simulink model "Comparison_SmithPredictor_MIAC_V4"  (R2018b)
settings: Solver=FixedStepDiscrete  StartTime=0.0  StopTime=15  FixedStep=1  RelTol=1e-3
libraries: simulink x2, slident x2
settings Model: Creator=Trips  LastModifiedBy=Trips
settings ConfigComp: PLC_OutputDir=Generated_V4  PLC_TargetIDE=step7  PLC_GenerateReport=off  PLC_LaunchReport=off

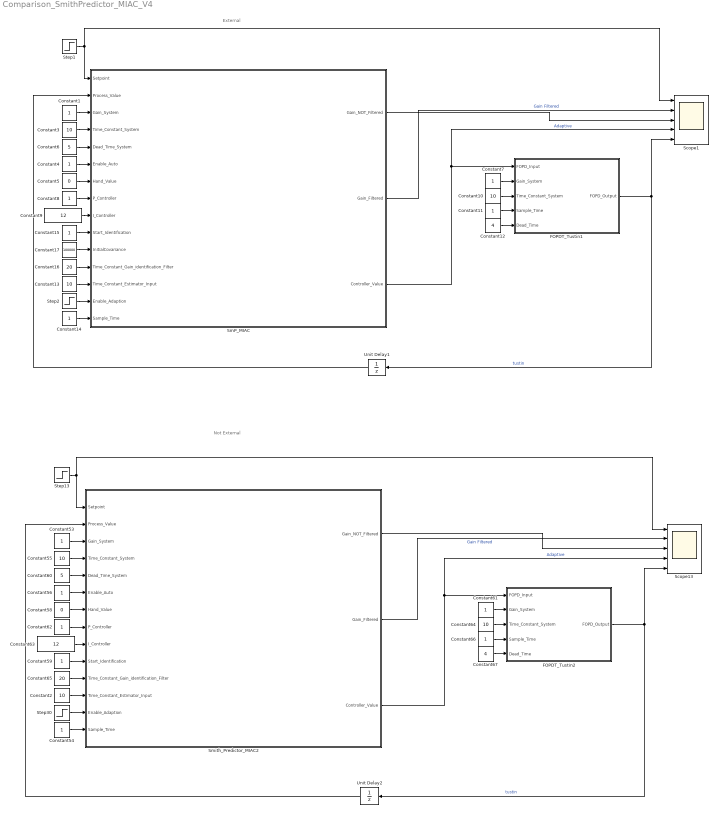
== system Comparison_SmithPredictor_MIAC_V4 ==
  note: External
  note: Not External
  Constant{1,4,7..8,11,14..15,53..54,56,59,61..62,66} (14 alike) : Constant
  Constant{2..3,10,13,55,64} (6 alike) : Constant  Value=10
  Constant12 : Constant  Value=4
  Constant16 : Constant  Value=20
  Constant17 : Constant  Value=100000
  Constant5 : Constant  Value=0
  Constant58 : Constant  Value=0
  Constant6 : Constant  Value=5
  Constant60 : Constant  Value=5
  Constant63 : Constant  Value=12
  Constant65 : Constant  Value=20
  Constant67 : Constant  Value=4
  Constant9 : Constant  Value=12
  FOPDT_Tustin1 : Subsystem  TreatAsAtomicUnit=on  SystemSampleTime=1
  FOPDT_Tustin2 : Subsystem  TreatAsAtomicUnit=on  SystemSampleTime=1
  Scope1 : Scope  NumInputPorts=5
  Scope13 : Scope  NumInputPorts=5
  SmP_MIAC : Subsystem  TreatAsAtomicUnit=on  SystemSampleTime=1
  Smith_Predictor_MIAC2 : Subsystem  TreatAsAtomicUnit=on  SystemSampleTime=1
  Step1 : Step  After=3  SampleTime=0
  Step13 : Step  After=3  SampleTime=0
  Step2 : Step  Time=500  After=0  SampleTime=0
  Step30 : Step  Time=500  After=0  SampleTime=0
  Unit Delay1 : UnitDelay  SampleTime=-1
  Unit Delay2 : UnitDelay  SampleTime=-1
  wires:
  Smith_Predictor_MIAC2/3(Controller_Value) -> Scope13/4, FOPDT_Tustin2/1(FOPD_Input)  "Adaptive"
  Constant56/1 -> Smith_Predictor_MIAC2/6(" Enable_Auto")
  Constant60/1 -> Smith_Predictor_MIAC2/5(Dead_Time_System)
  Constant62/1 -> Smith_Predictor_MIAC2/8(P_Controller)
  Constant55/1 -> Smith_Predictor_MIAC2/4(Time_Constant_System)
  Unit Delay2/1 -> Smith_Predictor_MIAC2/2(Process_Value)
  Constant58/1 -> Smith_Predictor_MIAC2/7(Hand_Value)
  Constant2/1 -> Smith_Predictor_MIAC2/12(Time_Constant_Estimator_Input)
  Constant63/1 -> Smith_Predictor_MIAC2/9(I_Controller)
  Constant65/1 -> Smith_Predictor_MIAC2/11(Time_Constant_Gain_identification_Filter)
  Constant66/1 -> FOPDT_Tustin2/4(Sample_Time)
  Constant61/1 -> FOPDT_Tustin2/2(Gain_System)
  Constant67/1 -> FOPDT_Tustin2/5(" Dead_Time")
  Constant64/1 -> FOPDT_Tustin2/3(Time_Constant_System)
  Step13/1 -> Smith_Predictor_MIAC2/1(Setpoint), Scope13/1
  FOPDT_Tustin2/1(FOPD_Output) -> Scope13/5, Unit Delay2/1  "tustin"
  Smith_Predictor_MIAC2/2(Gain_Filtered) -> Scope13/2  "Gain Filtered"
  Constant54/1 -> Smith_Predictor_MIAC2/14(Sample_Time)
  Constant53/1 -> Smith_Predictor_MIAC2/3(Gain_System)
  Smith_Predictor_MIAC2/1(Gain_NOT_Filtered) -> Scope13/3
  Step30/1 -> Smith_Predictor_MIAC2/13(Enable_Adaption)
  Constant59/1 -> Smith_Predictor_MIAC2/10(Start_Identification)
  SmP_MIAC/1(Gain_NOT_Filtered) -> Scope1/3
  Constant1/1 -> SmP_MIAC/3(Gain_System)
  SmP_MIAC/2(Gain_Filtered) -> Scope1/2  "Gain Filtered"
  Step1/1 -> SmP_MIAC/1(Setpoint), Scope1/1
  Constant10/1 -> FOPDT_Tustin1/3(Time_Constant_System)
  Constant12/1 -> FOPDT_Tustin1/5(" Dead_Time")
  Constant7/1 -> FOPDT_Tustin1/2(Gain_System)
  Constant11/1 -> FOPDT_Tustin1/4(Sample_Time)
  Constant3/1 -> SmP_MIAC/4(Time_Constant_System)
  Constant5/1 -> SmP_MIAC/7(Hand_Value)
  Constant8/1 -> SmP_MIAC/8(P_Controller)
  Unit Delay1/1 -> SmP_MIAC/2(Process_Value)
  Constant6/1 -> SmP_MIAC/5(Dead_Time_System)
  Constant4/1 -> SmP_MIAC/6(" Enable_Auto")
  FOPDT_Tustin1/1(FOPD_Output) -> Scope1/5, Unit Delay1/1  "tustin"
  SmP_MIAC/3(Controller_Value) -> Scope1/4, FOPDT_Tustin1/1(FOPD_Input)  "Adaptive"
  Constant9/1 -> SmP_MIAC/9(I_Controller)
  Step2/1 -> SmP_MIAC/14(Enable_Adaption)
  Constant14/1 -> SmP_MIAC/15(Sample_Time)
  Constant16/1 -> SmP_MIAC/12(Time_Constant_Gain_identification_Filter)
  Constant15/1 -> SmP_MIAC/10(Start_Identification)
  Constant13/1 -> SmP_MIAC/13(Time_Constant_Estimator_Input)
  Constant17/1 -> SmP_MIAC/11(InitialCovariance)

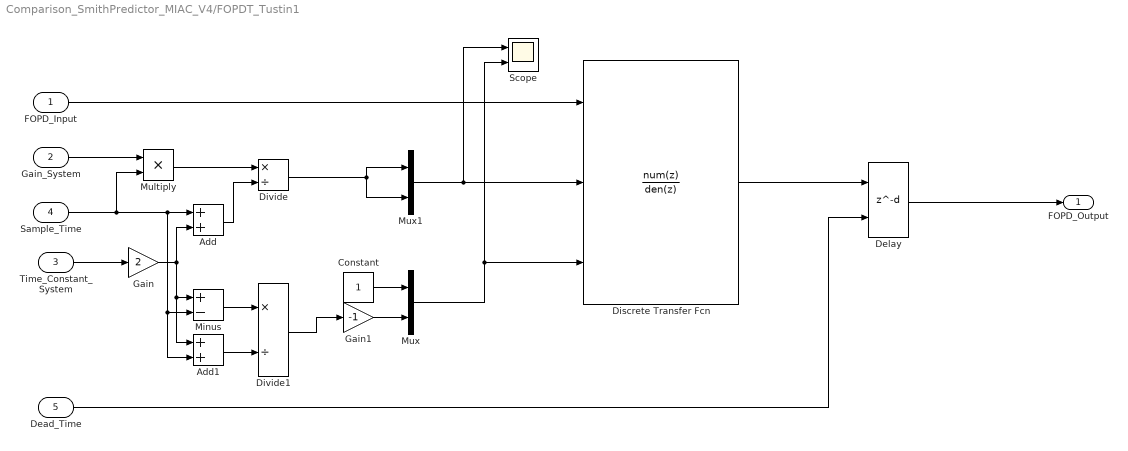
== system Comparison_SmithPredictor_MIAC_V4/FOPDT_Tustin1 ==
  FOPD_Input : Inport
  Gain_System : Inport  Port=2
  Time_Constant_System : Inport  Port=3
  Sample_Time : Inport  Port=4
  " Dead_Time" : Inport  Port=5
  Add : Sum
  Add1 : Sum
  Constant : Constant
  Delay : Delay  DelayLengthSource=Input port  DelayLength=600  DelayLengthUpperLimit=800
      settings: InputPortMap=u0,p1
  Discrete Transfer Fcn : DiscreteTransferFcn  NumeratorSource=Input port  DenominatorSource=Input port  SampleTime=1  a0EqualsOne=on
      settings: InputPortMap=u0,p1,p3
  Divide : Product  Inputs=*/
  Divide1 : Product  Inputs=*/
  Gain : Gain  Gain=2
  Gain1 : Gain  Gain=-1
  Minus : Sum  Inputs=+-
  Multiply : Product
  Mux : Mux  Inputs=2
  Mux1 : Mux  Inputs=2
  Scope : Scope  NumInputPorts=2
  FOPD_Output : Outport
  wires:
  FOPD_Input/1 -> Discrete Transfer Fcn/1
  Discrete Transfer Fcn/1 -> Delay/1
  Mux/1 -> Scope/2, Discrete Transfer Fcn/3
  " Dead_Time"/1 -> Delay/2
  Sample_Time/1 -> Add1/2, Minus/2, Add/1, Multiply/2
  Mux1/1 -> Scope/1, Discrete Transfer Fcn/2
  Time_Constant_System/1 -> Gain/1
  Delay/1 -> FOPD_Output/1
  Gain_System/1 -> Multiply/1
  Multiply/1 -> Divide/1
  Gain/1 -> Add1/1, Minus/1, Add/2
  Add/1 -> Divide/2
  Divide/1 -> Mux1/2, Mux1/1
  Constant/1 -> Mux/1
  Minus/1 -> Divide1/1
  Add1/1 -> Divide1/2
  Divide1/1 -> Gain1/1
  Gain1/1 -> Mux/2

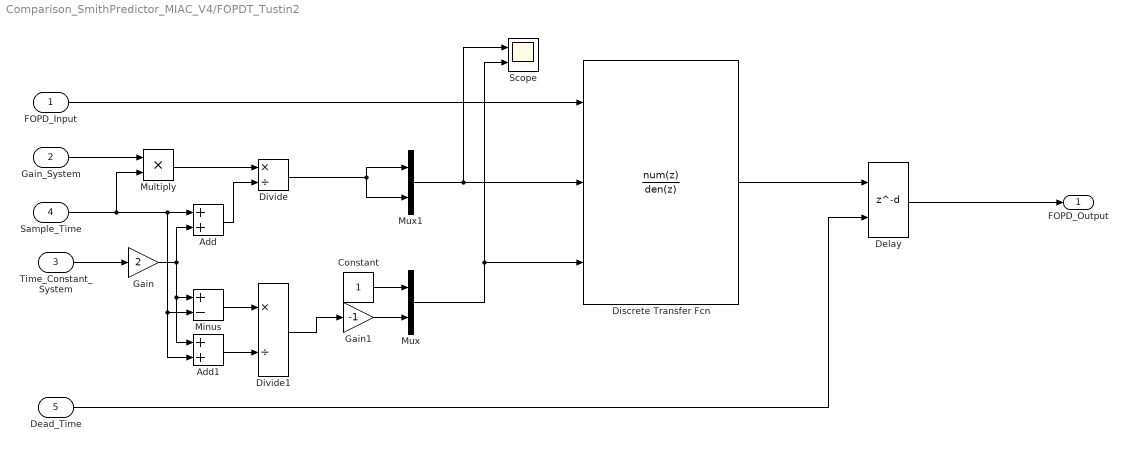
== system Comparison_SmithPredictor_MIAC_V4/FOPDT_Tustin2 ==
  FOPD_Input : Inport
  Gain_System : Inport  Port=2
  Time_Constant_System : Inport  Port=3
  Sample_Time : Inport  Port=4
  " Dead_Time" : Inport  Port=5
  Add : Sum
  Add1 : Sum
  Constant : Constant
  Delay : Delay  DelayLengthSource=Input port  DelayLength=600  DelayLengthUpperLimit=800
      settings: InputPortMap=u0,p1
  Discrete Transfer Fcn : DiscreteTransferFcn  NumeratorSource=Input port  DenominatorSource=Input port  SampleTime=1  a0EqualsOne=on
      settings: InputPortMap=u0,p1,p3
  Divide : Product  Inputs=*/
  Divide1 : Product  Inputs=*/
  Gain : Gain  Gain=2
  Gain1 : Gain  Gain=-1
  Minus : Sum  Inputs=+-
  Multiply : Product
  Mux : Mux  Inputs=2
  Mux1 : Mux  Inputs=2
  Scope : Scope  NumInputPorts=2
  FOPD_Output : Outport
  wires:
  FOPD_Input/1 -> Discrete Transfer Fcn/1
  Discrete Transfer Fcn/1 -> Delay/1
  Mux/1 -> Scope/2, Discrete Transfer Fcn/3
  " Dead_Time"/1 -> Delay/2
  Sample_Time/1 -> Add1/2, Minus/2, Add/1, Multiply/2
  Mux1/1 -> Scope/1, Discrete Transfer Fcn/2
  Time_Constant_System/1 -> Gain/1
  Delay/1 -> FOPD_Output/1
  Gain_System/1 -> Multiply/1
  Multiply/1 -> Divide/1
  Gain/1 -> Add1/1, Minus/1, Add/2
  Add/1 -> Divide/2
  Divide/1 -> Mux1/2, Mux1/1
  Constant/1 -> Mux/1
  Minus/1 -> Divide1/1
  Add1/1 -> Divide1/2
  Divide1/1 -> Gain1/1
  Gain1/1 -> Mux/2

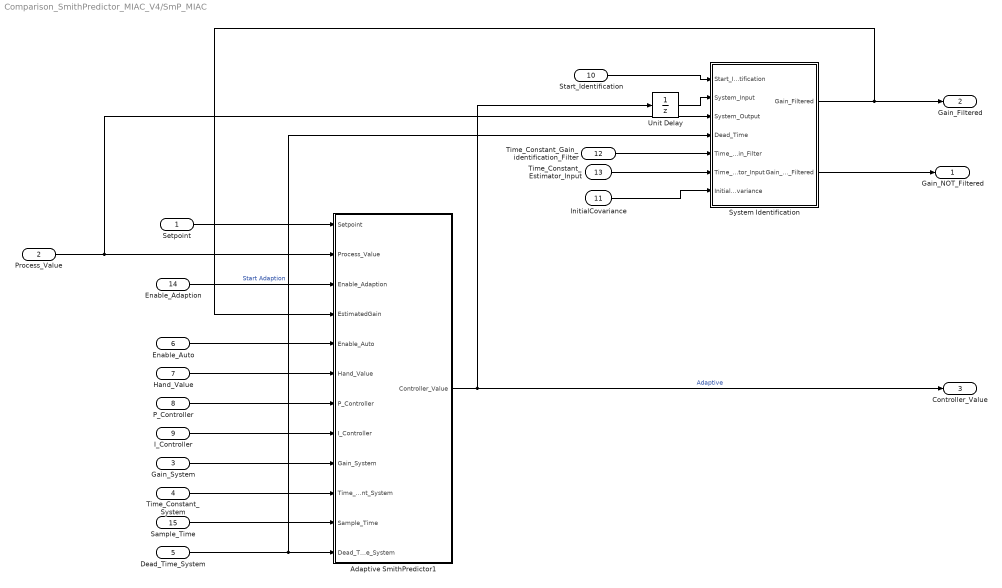
== system Comparison_SmithPredictor_MIAC_V4/SmP_MIAC ==
  Setpoint : Inport
  Process_Value : Inport  Port=2
  Gain_System : Inport  Port=3
  Time_Constant_System : Inport  Port=4
  Dead_Time_System : Inport  Port=5
  " Enable_Auto" : Inport  Port=6
  Hand_Value : Inport  Port=7
  P_Controller : Inport  Port=8
  I_Controller : Inport  Port=9
  Start_Identification : Inport  Port=10  PortDimensions=1  SampleTime=1
  InitialCovariance : Inport  Port=11
  Time_Constant_Gain_identification_Filter : Inport  Port=12
  Time_Constant_Estimator_Input : Inport  Port=13
  Enable_Adaption : Inport  Port=14
  Sample_Time : Inport  Port=15
  Adaptive SmithPredictor1 : Subsystem  TreatAsAtomicUnit=on  SystemSampleTime=1
  System Identification : Subsystem  TreatAsAtomicUnit=on  SystemSampleTime=1
  Unit Delay : UnitDelay
  Gain_NOT_Filtered : Outport
  Gain_Filtered : Outport  Port=2
  Controller_Value : Outport  Port=3
  wires:
  Gain_System/1 -> Adaptive SmithPredictor1/9(Gain_System)
  Dead_Time_System/1 -> Adaptive SmithPredictor1/12(" Dead_Time_System"), System Identification/4(Dead_Time)
  Adaptive SmithPredictor1/1(Controller_Value) -> Unit Delay/1, Controller_Value/1  "Adaptive"
  Time_Constant_System/1 -> Adaptive SmithPredictor1/10(Time_Constant_System)
  P_Controller/1 -> Adaptive SmithPredictor1/7(P_Controller)
  Sample_Time/1 -> Adaptive SmithPredictor1/11(Sample_Time)
  I_Controller/1 -> Adaptive SmithPredictor1/8(I_Controller)
  Enable_Adaption/1 -> Adaptive SmithPredictor1/3(Enable_Adaption)  "Start Adaption"
  System Identification/2(Gain_Not_Filtered) -> Gain_NOT_Filtered/1
  Setpoint/1 -> Adaptive SmithPredictor1/1(Setpoint)
  Start_Identification/1 -> System Identification/1(Start_Identification)
  System Identification/1(Gain_Filtered) -> Gain_Filtered/1, Adaptive SmithPredictor1/4(EstimatedGain)
  " Enable_Auto"/1 -> Adaptive SmithPredictor1/5(Enable_Auto)
  Hand_Value/1 -> Adaptive SmithPredictor1/6(Hand_Value)
  Process_Value/1 -> System Identification/3(System_Output), Adaptive SmithPredictor1/2(Process_Value)
  Unit Delay/1 -> System Identification/2(System_Input)
  Time_Constant_Gain_identification_Filter/1 -> System Identification/5(Time_Constant_Gain_Filter)
  Time_Constant_Estimator_Input/1 -> System Identification/6(Time_Constant_Estimator_Input)
  InitialCovariance/1 -> System Identification/7(InitialCovariance)

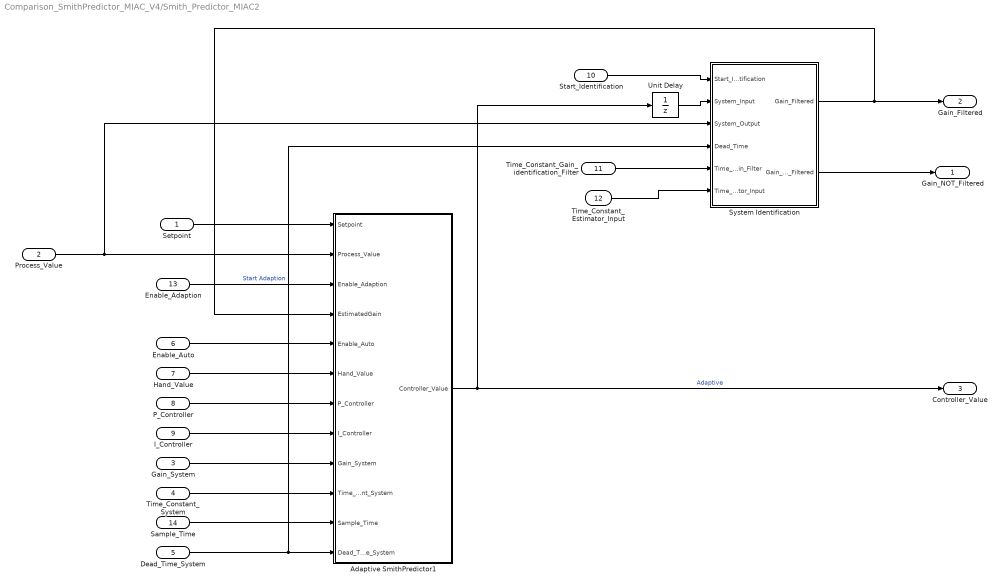
== system Comparison_SmithPredictor_MIAC_V4/Smith_Predictor_MIAC2 ==
  Setpoint : Inport
  Process_Value : Inport  Port=2
  Gain_System : Inport  Port=3
  Time_Constant_System : Inport  Port=4
  Dead_Time_System : Inport  Port=5
  " Enable_Auto" : Inport  Port=6
  Hand_Value : Inport  Port=7
  P_Controller : Inport  Port=8
  I_Controller : Inport  Port=9
  Start_Identification : Inport  Port=10  PortDimensions=1  SampleTime=1
  Time_Constant_Gain_identification_Filter : Inport  Port=11
  Time_Constant_Estimator_Input : Inport  Port=12
  Enable_Adaption : Inport  Port=13
  Sample_Time : Inport  Port=14
  Adaptive SmithPredictor1 : Subsystem  TreatAsAtomicUnit=on  SystemSampleTime=1
  System Identification : Subsystem  TreatAsAtomicUnit=on  SystemSampleTime=1
  Unit Delay : UnitDelay
  Gain_NOT_Filtered : Outport
  Gain_Filtered : Outport  Port=2
  Controller_Value : Outport  Port=3
  wires:
  Gain_System/1 -> Adaptive SmithPredictor1/9(Gain_System)
  Dead_Time_System/1 -> Adaptive SmithPredictor1/12(" Dead_Time_System"), System Identification/4(Dead_Time)
  Adaptive SmithPredictor1/1(Controller_Value) -> Unit Delay/1, Controller_Value/1  "Adaptive"
  Time_Constant_System/1 -> Adaptive SmithPredictor1/10(Time_Constant_System)
  P_Controller/1 -> Adaptive SmithPredictor1/7(P_Controller)
  Sample_Time/1 -> Adaptive SmithPredictor1/11(Sample_Time)
  I_Controller/1 -> Adaptive SmithPredictor1/8(I_Controller)
  Enable_Adaption/1 -> Adaptive SmithPredictor1/3(Enable_Adaption)  "Start Adaption"
  System Identification/2(Gain_Not_Filtered) -> Gain_NOT_Filtered/1
  Setpoint/1 -> Adaptive SmithPredictor1/1(Setpoint)
  Start_Identification/1 -> System Identification/1(Start_Identification)
  System Identification/1(Gain_Filtered) -> Gain_Filtered/1, Adaptive SmithPredictor1/4(EstimatedGain)
  " Enable_Auto"/1 -> Adaptive SmithPredictor1/5(Enable_Auto)
  Hand_Value/1 -> Adaptive SmithPredictor1/6(Hand_Value)
  Process_Value/1 -> System Identification/3(System_Output), Adaptive SmithPredictor1/2(Process_Value)
  Unit Delay/1 -> System Identification/2(System_Input)
  Time_Constant_Gain_identification_Filter/1 -> System Identification/5(Time_Constant_Gain_Filter)
  Time_Constant_Estimator_Input/1 -> System Identification/6(Time_Constant_Estimator_Input)

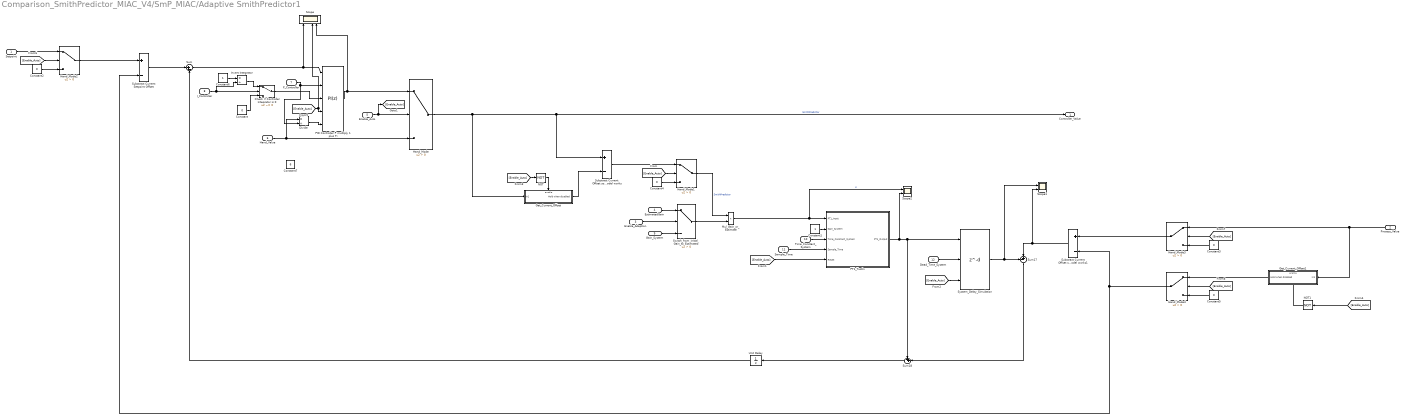
== system Comparison_SmithPredictor_MIAC_V4/SmP_MIAC/Adaptive SmithPredictor1 ==
  Setpoint : Inport
  Process_Value : Inport  Port=2
  Enable_Adaption : Inport  Port=3
  EstimatedGain : Inport  Port=4
  Enable_Auto : Inport  Port=5
  Hand_Value : Inport  Port=6
  P_Controller : Inport  Port=7
  I_Controller : Inport  Port=8
  Gain_System : Inport  Port=9
  Time_Constant_System : Inport  Port=10
  Sample_Time : Inport  Port=11
  " Dead_Time_System" : Inport  Port=12
  Check if Controller Integrator is 0 : Switch  Criteria=u2 ~= 0
  Constant{,2..5} (5 alike) : Constant  Value=0
  Constant1 : Constant
  Constant6 : Constant
  Constant7 : Constant  Value=6
  Divide : Product  Inputs=*/
  Get_Current_Offset : Subsystem
  Get_Current_Offset1 : Subsystem
  Hand_Mode{,1..4} (5 alike) : Switch  Criteria=u2 > Threshold
  Invert Integrator : Product  Inputs=*/
  Mul_Gain_or_Estimate : Product
  NOT : Logic  Operator=NOT  IconShape=distinctive  AllPortsSameDT=off  OutDataTypeStr=boolean
  NOT1 : Logic  Operator=NOT  IconShape=distinctive  AllPortsSameDT=off  OutDataTypeStr=boolean
  "PID Controller P multiply 1 plus Ti " : simulink/Continuous/PID Controller  Controller=PI  Form=Ideal  TimeDomain=Discrete-time  SampleTime=1  IntegratorMethod=Forward Euler  FilterMethod=Forward Euler  ControllerParametersSource=external  P=3.04732259067536  I=0.00445689106465138  D=118.272348286844  UseFilter=on  N=0.00420306193364532  TunerSelectOption=Transfer Function Based (PID Tuner App)  InitialConditionSource=external  InitialConditionForIntegrator=0  InitialConditionForFilter=0  DifferentiatorICPrevScaledInput=0  ExternalReset=rising  TrackingMode=off  Kt=1  LimitOutput=on  UpperSaturationLimit=100  LowerSaturationLimit=0  LinearizeAsGain=on  AntiWindupMode=none  Kb=1  POutMin=[]  POutMax=[]  IOutMin=[]  IOutMax=[]  DOutMin=[]  DOutMax=[]  NOutMin=[]  NOutMax=[]  SumOutMin=[]  SumOutMax=[]  SaturationOutMin=[]  SaturationOutMax=[]  PParamMin=[]  PParamMax=[]  IParamMin=[]  IParamMax=[]  DParamMin=[]  DParamMax=[]  NParamMin=[]  NParamMax=[]  KbParamMin=[]  KbParamMax=[]  KtParamMin=[]  KtParamMax=[]  KbOutMin=[]  KbOutMax=[]  KtOutMin=[]  KtOutMax=[]  IntegratorOutMin=[]  IntegratorOutMax=[]  FilterOutMin=[]  FilterOutMax=[]  SumI1OutMin=[]  SumI1OutMax=[]  SumI2OutMin=[]  SumI2OutMax=[]  SumI3OutMin=[]  SumI3OutMax=[]  SumI4OutMin=[]  SumI4OutMax=[]  SumDOutMin=[]  SumDOutMax=[]  DifferentiatorOutMin=[]  DifferentiatorOutMax=[]  FilterDiffOutCoefMin=[]  FilterDiffOutCoefMax=[]  ReciprocalOutMin=[]  ReciprocalOutMax=[]  SumDenOutMin=[]  SumDenOutMax=[]  SumNumOutMin=[]  SumNumOutMax=[]  DivideOutMin=[]  DivideOutMax=[]  IntegratorContinuousStateAttributes=''  IntegratorStateMustResolveToSignalObject=off  IntegratorRTWStateStorageClass=Auto  FilterContinuousStateAttributes=''  FilterStateMustResolveToSignalObject=off  FilterRTWStateStorageClass=Auto  ParallelPVariant=Passthrough  IdealPVariant=ExternalParameters  IVariant=ExternalParameters  DVariant=Disabled  IntegratorVariant=Discrete  SatVariant=Enabled  AWVariant=Passthrough  PCopyVariant=Disabled  TRVariant=Disabled  FdbkBlocksVariant=Forward  IdealPFdbkVariant=Disabled  SatFdbkVariant=Disabled  DerivativeFilterVariant=Disabled  NVariant=Disabled  NCopyVariant=Disabled_SignalSpec  FilterICVariant=Disabled  IntegratorICVariant=ExternalICs  ExternalResetVariant=ExternalReset  TRSumVariant=Passthrough  SumFdbkVariant=Disabled  SumVariant=Sum_PI
  PT1_Tustin : Subsystem  TreatAsAtomicUnit=on  SystemSampleTime=1
  Scope : Scope  NumInputPorts=4
  Scope1 : Scope  NumInputPorts=2
  Scope2 : Scope  NumInputPorts=2
  Substract Current Offset so that the linearised model works : Sum  Inputs=+-
  Substract Current Offset so that the linearised model works1 : Sum  Inputs=+-
  Substract Current Setpoint Offset : Sum  Inputs=+-
  Sum : Sum  Inputs=|+-
  Sum17 : Sum  Inputs=-+|
  Sum18 : Sum  Inputs=++|
  Switch_from_initial_Gain_to_Estimated : Switch  Criteria=u2 > Threshold
  System_Delay_Simulation : Delay  DelayLengthSource=Input port  DelayLength=600  DelayLengthUpperLimit=900  ExternalReset=Rising  SampleTime=1
      settings: InputPortMap=u0,p1,r5
  Unit Delay : UnitDelay
  Controller_Value : Outport
  wires:
  Substract Current Setpoint Offset/1 -> Sum/1
  Sum/1 -> "PID Controller P multiply 1 plus Ti "/1, Scope/1
  Hand_Mode/1 -> Get_Current_Offset/1(In1), Controller_Value/1, Substract Current Offset so that the linearised model works/1  "SmithPredictor"
  Substract Current Offset so that the linearised model works1/1 -> Scope1/2, Sum17/2
  PT1_Tustin/1(PT1_Output) -> Scope2/2, Sum18/1, System_Delay_Simulation/1
  System_Delay_Simulation/1 -> Scope1/1, Sum17/1
  Sum17/1 -> Sum18/2
  Mul_Gain_or_Estimate/1 -> Scope2/1, PT1_Tustin/1(PT1_Input)  "U"
  Switch_from_initial_Gain_to_Estimated/1 -> Mul_Gain_or_Estimate/2
  "PID Controller P multiply 1 plus Ti "/1 -> Hand_Mode/1, Scope/4
  Hand_Value/1 -> Divide/1, Hand_Mode/3
  Enable_Auto/1 -> [Enable_Auto], Hand_Mode/2
  P_Controller/1 -> "PID Controller P multiply 1 plus Ti "/2, Divide/2
  Check if Controller Integrator is 0/1 -> "PID Controller P multiply 1 plus Ti "/3
  " Dead_Time_System"/1 -> System_Delay_Simulation/2
  Gain_System/1 -> Switch_from_initial_Gain_to_Estimated/3
  Enable_Adaption/1 -> Switch_from_initial_Gain_to_Estimated/2
  EstimatedGain/1 -> Switch_from_initial_Gain_to_Estimated/1
  [Enable_Auto] -> Hand_Mode1/2
  Hand_Mode1/1 -> Mul_Gain_or_Estimate/1  "SmithPredictor"
  Constant4/1 -> Hand_Mode1/3
  [Enable_Auto] -> PT1_Tustin/5(Reset)
  [Enable_Auto] -> System_Delay_Simulation/3
  Substract Current Offset so that the linearised model works/1 -> Hand_Mode1/1
  Get_Current_Offset/1(Hold when disabled) -> Substract Current Offset so that the linearised model works/2
  [Enable_Auto] -> NOT/1
  NOT/1 -> Get_Current_Offset/Enable
  Sum18/1 -> Unit Delay/1
  Hand_Mode2/1 -> Substract Current Setpoint Offset/1
  NOT1/1 -> Get_Current_Offset1/Enable
  [Enable_Auto] -> NOT1/1
  Hand_Mode4/1 -> Substract Current Setpoint Offset/2, Substract Current Offset so that the linearised model works1/2
  Setpoint/1 -> Hand_Mode2/1
  [Enable_Auto] -> Hand_Mode2/2
  Constant2/1 -> Hand_Mode2/3
  Process_Value/1 -> Get_Current_Offset1/1(In1), Hand_Mode3/1
  [Enable_Auto] -> Hand_Mode3/2
  Constant3/1 -> Hand_Mode3/3
  Hand_Mode3/1 -> Substract Current Offset so that the linearised model works1/1
  Constant5/1 -> Hand_Mode4/3
  [Enable_Auto] -> Hand_Mode4/2
  Get_Current_Offset1/1(Hold when disabled) -> Hand_Mode4/1
  Time_Constant_System/1 -> PT1_Tustin/3(Time_Constant_System)
  Constant1/1 -> PT1_Tustin/2(Gain_System)
  Sample_Time/1 -> PT1_Tustin/4(Sample_Time)
  I_Controller/1 -> Check if Controller Integrator is 0/2, Invert Integrator/2
  Constant/1 -> Check if Controller Integrator is 0/3
  Invert Integrator/1 -> Check if Controller Integrator is 0/1
  Constant6/1 -> Invert Integrator/1
  Unit Delay/1 -> Sum/2
  [Enable_Auto] -> Scope/3, "PID Controller P multiply 1 plus Ti "/4
  Divide/1 -> "PID Controller P multiply 1 plus Ti "/5

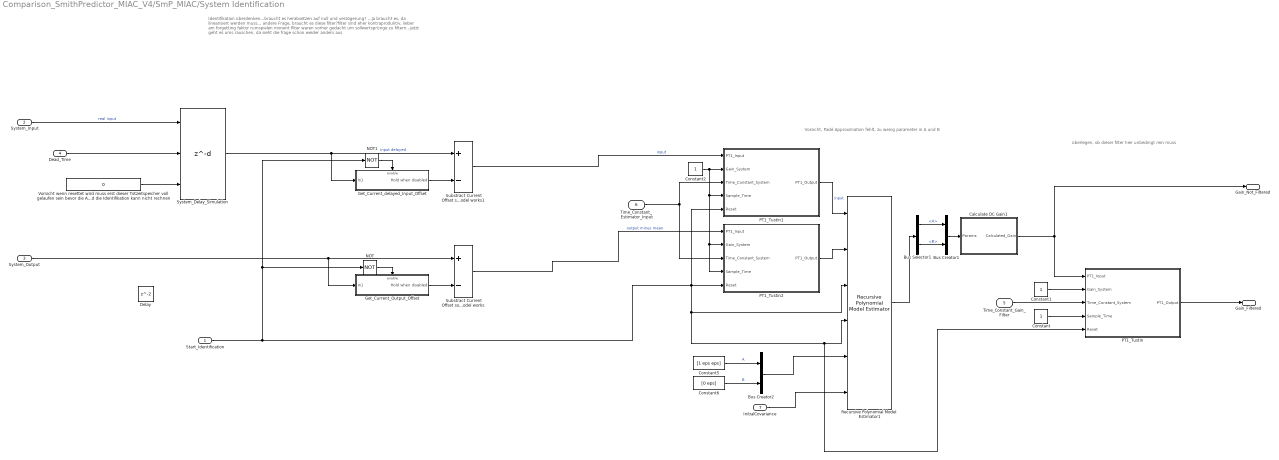
== system Comparison_SmithPredictor_MIAC_V4/SmP_MIAC/System Identification ==
  note: Vorsicht, Padé Approximation fehlt, zu wenig parameter in A und B
  note: überlegen, ob dieser filter hier unbedingt rein muss
  note: Identifikation überdenken...braucht es herabsetzen auf null und verzögerung?
      | ...ja braucht es, da linearisiert werden muss...
      |
      | andere Frage, braucht es diese filter?filter sind eher kontraproduktiv, lieber am forgetting faktor rumspielen
      | monent fliter waren vorher gedacht um sollwertsprünge zu filtern...jetzt geht es ums rauschen, da sieht die frage schon weider anders aus
  Start_Identification : Inport  SampleTime=1
  System_Input : Inport  Port=2
  System_Output : Inport  Port=3  SampleTime=1
  Dead_Time : Inport  Port=4
  Time_Constant_Gain_Filter : Inport  Port=5
  Time_Constant_Estimator_Input : Inport  Port=6
  InitialCovariance : Inport  Port=7  SampleTime=1
  Bus Creator1 : BusCreator  Inputs=2
  Bus Creator2 : BusCreator  Inputs=2
  Bus Selector1 : BusSelector  OutputSignals=A,B
  Calculate DC Gain1 : Subsystem  TreatAsAtomicUnit=on  SystemSampleTime=1
  Constant : Constant
  Constant1 : Constant
  Constant2 : Constant
  Constant5 : Constant  Value=[1 eps eps]  VectorParams1D=off
  Constant6 : Constant  Value=[0 eps]  VectorParams1D=off
  Delay : Delay
  Get_Current_Output_Offset : Subsystem
  Get_Current_delayed_Input_Offset : Subsystem
  NOT : Logic  Operator=NOT  IconShape=distinctive  AllPortsSameDT=off  OutDataTypeStr=boolean
  NOT1 : Logic  Operator=NOT  IconShape=distinctive  AllPortsSameDT=off  OutDataTypeStr=boolean
  PT1_Tustin : Subsystem  TreatAsAtomicUnit=on  SystemSampleTime=1
  PT1_Tustin1 : Subsystem  TreatAsAtomicUnit=on  SystemSampleTime=1
  PT1_Tustin2 : Subsystem  TreatAsAtomicUnit=on  SystemSampleTime=1
  Recursive Polynomial Model Estimator1 : slident/Estimators/Recursive Polynomial Model Estimator  ModelStructure=ARX  InitialEstimateSource=External  A0=2  B0=1  C0=1  D0=1  F0=1  nk=1  P0=10  InitialInputs=0  InitialOutputs=0  History=Infinite  WindowLength=2000  EstimationMethod=Forgetting Factor  AdaptationParameter=1  HasTimeVaryingAdaptationParameter=off  NormalizationBias=eps  OutputError=off  OutputP=off  AddEnablePort=on  ExternalReset=Rising  InputProcessing=Sample-based  Ts=1
      settings: SourceProductName=System Identification Toolbox  SourceProductBaseCode=ID
  Substract Current Offset so that the linearised model works : Sum  Inputs=+-
  Substract Current Offset so that the linearised model works1 : Sum  Inputs=+-
  System_Delay_Simulation : Delay  DelayLengthSource=Input port  DelayLength=600  DelayLengthUpperLimit=900  ExternalReset=Rising  SampleTime=1
      settings: InputPortMap=u0,p1,r5
  Vorsicht wenn resettet wird muss erst dieser Totzeitspeicher voll gelaufen sein bevor die Adaption starten darf Sonst kommt heir immer 0 raus und die Identifikation kann nicht rechnen : Constant  Value=0
  Gain_Filtered : Outport
  Gain_Not_Filtered : Outport  Port=2
  wires:
  Recursive Polynomial Model Estimator1/1 -> Bus Selector1/1
  Substract Current Offset so that the linearised model works1/1 -> PT1_Tustin1/1(PT1_Input)  "input"
  Bus Creator1/1 -> Calculate DC Gain1/1(Params)
  Bus Selector1/1 -> Bus Creator1/1  "<A>"
  Bus Selector1/2 -> Bus Creator1/2  "<B>"
  Substract Current Offset so that the linearised model works/1 -> PT1_Tustin2/1(PT1_Input)  "output minus mean"
  NOT/1 -> Get_Current_Output_Offset/Enable
  Get_Current_Output_Offset/1(Hold when disabled) -> Substract Current Offset so that the linearised model works/2
  System_Output/1 -> Get_Current_Output_Offset/1(In1), Substract Current Offset so that the linearised model works/1
  Get_Current_delayed_Input_Offset/1(Hold when disabled) -> Substract Current Offset so that the linearised model works1/2
  NOT1/1 -> Get_Current_delayed_Input_Offset/Enable
  PT1_Tustin/1(PT1_Output) -> Gain_Filtered/1
  System_Input/1 -> System_Delay_Simulation/1  "real input"
  Vorsicht wenn resettet wird muss erst dieser Totzeitspeicher voll gelaufen sein bevor die Adaption starten darf Sonst kommt heir immer 0 raus und die Identifikation kann nicht rechnen/1 -> System_Delay_Simulation/3
  Dead_Time/1 -> System_Delay_Simulation/2
  System_Delay_Simulation/1 -> Substract Current Offset so that the linearised model works1/1, Get_Current_delayed_Input_Offset/1(In1)  "input delayed"
  Calculate DC Gain1/1(Calculated_Gain) -> PT1_Tustin/1(PT1_Input), Gain_Not_Filtered/1
  Start_Identification/1 -> NOT/1, NOT1/1, PT1_Tustin2/5(Reset), Recursive Polynomial Model Estimator1/3, PT1_Tustin/5(Reset), Recursive Polynomial Model Estimator1/4, PT1_Tustin1/5(Reset)
  Constant/1 -> PT1_Tustin/4(Sample_Time)
  Constant1/1 -> PT1_Tustin/2(Gain_System)
  Time_Constant_Gain_Filter/1 -> PT1_Tustin/3(Time_Constant_System)
  PT1_Tustin1/1(PT1_Output) -> Recursive Polynomial Model Estimator1/1  "input"
  PT1_Tustin2/1(PT1_Output) -> Recursive Polynomial Model Estimator1/2
  Constant2/1 -> PT1_Tustin1/2(Gain_System), PT1_Tustin2/2(Gain_System), PT1_Tustin2/4(Sample_Time), PT1_Tustin1/4(Sample_Time)
  Time_Constant_Estimator_Input/1 -> PT1_Tustin2/3(Time_Constant_System), PT1_Tustin1/3(Time_Constant_System)
  Constant6/1 -> Bus Creator2/2  "B"
  Constant5/1 -> Bus Creator2/1  "A"
  Bus Creator2/1 -> Recursive Polynomial Model Estimator1/5
  InitialCovariance/1 -> Recursive Polynomial Model Estimator1/6

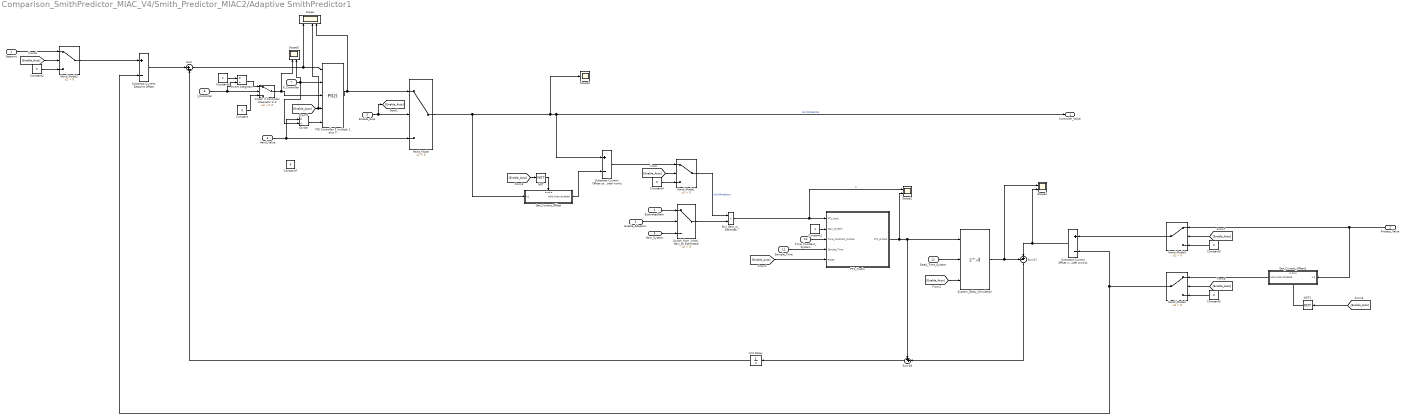
== system Comparison_SmithPredictor_MIAC_V4/Smith_Predictor_MIAC2/Adaptive SmithPredictor1 ==
  Setpoint : Inport
  Process_Value : Inport  Port=2
  Enable_Adaption : Inport  Port=3
  EstimatedGain : Inport  Port=4
  Enable_Auto : Inport  Port=5
  Hand_Value : Inport  Port=6
  P_Controller : Inport  Port=7
  I_Controller : Inport  Port=8
  Gain_System : Inport  Port=9
  Time_Constant_System : Inport  Port=10
  Sample_Time : Inport  Port=11
  " Dead_Time_System" : Inport  Port=12
  Check if Controller Integrator is 0 : Switch  Criteria=u2 ~= 0
  Constant{,2..5} (5 alike) : Constant  Value=0
  Constant1 : Constant
  Constant6 : Constant
  Constant7 : Constant  Value=6
  Divide : Product  Inputs=*/
  Get_Current_Offset : Subsystem
  Get_Current_Offset1 : Subsystem
  Hand_Mode{,1..4} (5 alike) : Switch  Criteria=u2 > Threshold
  Invert Integrator : Product  Inputs=*/
  Mul_Gain_or_Estimate : Product
  NOT : Logic  Operator=NOT  IconShape=distinctive  AllPortsSameDT=off  OutDataTypeStr=boolean
  NOT1 : Logic  Operator=NOT  IconShape=distinctive  AllPortsSameDT=off  OutDataTypeStr=boolean
  "PID Controller P multiply 1 plus Ti " : simulink/Continuous/PID Controller  Controller=PI  Form=Ideal  TimeDomain=Discrete-time  SampleTime=1  IntegratorMethod=Forward Euler  FilterMethod=Forward Euler  ControllerParametersSource=external  P=3.04732259067536  I=0.00445689106465138  D=118.272348286844  UseFilter=on  N=0.00420306193364532  TunerSelectOption=Transfer Function Based (PID Tuner App)  InitialConditionSource=external  InitialConditionForIntegrator=0  InitialConditionForFilter=0  DifferentiatorICPrevScaledInput=0  ExternalReset=rising  TrackingMode=off  Kt=1  LimitOutput=on  UpperSaturationLimit=100  LowerSaturationLimit=0  LinearizeAsGain=on  AntiWindupMode=none  Kb=1  POutMin=[]  POutMax=[]  IOutMin=[]  IOutMax=[]  DOutMin=[]  DOutMax=[]  NOutMin=[]  NOutMax=[]  SumOutMin=[]  SumOutMax=[]  SaturationOutMin=[]  SaturationOutMax=[]  PParamMin=[]  PParamMax=[]  IParamMin=[]  IParamMax=[]  DParamMin=[]  DParamMax=[]  NParamMin=[]  NParamMax=[]  KbParamMin=[]  KbParamMax=[]  KtParamMin=[]  KtParamMax=[]  KbOutMin=[]  KbOutMax=[]  KtOutMin=[]  KtOutMax=[]  IntegratorOutMin=[]  IntegratorOutMax=[]  FilterOutMin=[]  FilterOutMax=[]  SumI1OutMin=[]  SumI1OutMax=[]  SumI2OutMin=[]  SumI2OutMax=[]  SumI3OutMin=[]  SumI3OutMax=[]  SumI4OutMin=[]  SumI4OutMax=[]  SumDOutMin=[]  SumDOutMax=[]  DifferentiatorOutMin=[]  DifferentiatorOutMax=[]  FilterDiffOutCoefMin=[]  FilterDiffOutCoefMax=[]  ReciprocalOutMin=[]  ReciprocalOutMax=[]  SumDenOutMin=[]  SumDenOutMax=[]  SumNumOutMin=[]  SumNumOutMax=[]  DivideOutMin=[]  DivideOutMax=[]  IntegratorContinuousStateAttributes=''  IntegratorStateMustResolveToSignalObject=off  IntegratorRTWStateStorageClass=Auto  FilterContinuousStateAttributes=''  FilterStateMustResolveToSignalObject=off  FilterRTWStateStorageClass=Auto  ParallelPVariant=Passthrough  IdealPVariant=ExternalParameters  IVariant=ExternalParameters  DVariant=Disabled  IntegratorVariant=Discrete  SatVariant=Enabled  AWVariant=Passthrough  PCopyVariant=Disabled  TRVariant=Disabled  FdbkBlocksVariant=Forward  IdealPFdbkVariant=Disabled  SatFdbkVariant=Disabled  DerivativeFilterVariant=Disabled  NVariant=Disabled  NCopyVariant=Disabled_SignalSpec  FilterICVariant=Disabled  IntegratorICVariant=ExternalICs  ExternalResetVariant=ExternalReset  TRSumVariant=Passthrough  SumFdbkVariant=Disabled  SumVariant=Sum_PI
  PT1_Tustin : Subsystem  TreatAsAtomicUnit=on  SystemSampleTime=1
  Scope : Scope  NumInputPorts=4
  Scope1 : Scope  NumInputPorts=2
  Scope2 : Scope  NumInputPorts=2
  Scope3 : Scope  NumInputPorts=2
  Scope4 : Scope
  Substract Current Offset so that the linearised model works : Sum  Inputs=+-
  Substract Current Offset so that the linearised model works1 : Sum  Inputs=+-
  Substract Current Setpoint Offset : Sum  Inputs=+-
  Sum : Sum  Inputs=|+-
  Sum17 : Sum  Inputs=-+|
  Sum18 : Sum  Inputs=++|
  Switch_from_initial_Gain_to_Estimated : Switch  Criteria=u2 > Threshold
  System_Delay_Simulation : Delay  DelayLengthSource=Input port  DelayLength=600  DelayLengthUpperLimit=800  ExternalReset=Rising  SampleTime=1
      settings: InputPortMap=u0,p1,r5
  Unit Delay : UnitDelay
  Controller_Value : Outport
  wires:
  Substract Current Setpoint Offset/1 -> Sum/1
  Sum/1 -> "PID Controller P multiply 1 plus Ti "/1, Scope/1
  Hand_Mode/1 -> Get_Current_Offset/1(In1), Scope4/1, Controller_Value/1, Substract Current Offset so that the linearised model works/1  "SmithPredictor"
  Substract Current Offset so that the linearised model works1/1 -> Scope1/2, Sum17/2
  PT1_Tustin/1(PT1_Output) -> Scope2/2, Sum18/1, System_Delay_Simulation/1
  System_Delay_Simulation/1 -> Scope1/1, Sum17/1
  Sum17/1 -> Sum18/2
  Mul_Gain_or_Estimate/1 -> Scope2/1, PT1_Tustin/1(PT1_Input)  "U"
  Switch_from_initial_Gain_to_Estimated/1 -> Mul_Gain_or_Estimate/2
  "PID Controller P multiply 1 plus Ti "/1 -> Hand_Mode/1, Scope/4
  Hand_Value/1 -> Divide/1, Hand_Mode/3
  Enable_Auto/1 -> [Enable_Auto], Hand_Mode/2
  P_Controller/1 -> "PID Controller P multiply 1 plus Ti "/2, Scope3/2, Divide/2
  Check if Controller Integrator is 0/1 -> Scope3/1, "PID Controller P multiply 1 plus Ti "/3
  " Dead_Time_System"/1 -> System_Delay_Simulation/2
  Gain_System/1 -> Switch_from_initial_Gain_to_Estimated/3
  Enable_Adaption/1 -> Switch_from_initial_Gain_to_Estimated/2
  EstimatedGain/1 -> Switch_from_initial_Gain_to_Estimated/1
  [Enable_Auto] -> Hand_Mode1/2
  Hand_Mode1/1 -> Mul_Gain_or_Estimate/1  "SmithPredictor"
  Constant4/1 -> Hand_Mode1/3
  [Enable_Auto] -> PT1_Tustin/5(Reset)
  [Enable_Auto] -> System_Delay_Simulation/3
  Substract Current Offset so that the linearised model works/1 -> Hand_Mode1/1
  Get_Current_Offset/1(Hold when disabled) -> Substract Current Offset so that the linearised model works/2
  [Enable_Auto] -> NOT/1
  NOT/1 -> Get_Current_Offset/Enable
  Sum18/1 -> Unit Delay/1
  Hand_Mode2/1 -> Substract Current Setpoint Offset/1
  NOT1/1 -> Get_Current_Offset1/Enable
  [Enable_Auto] -> NOT1/1
  Hand_Mode4/1 -> Substract Current Setpoint Offset/2, Substract Current Offset so that the linearised model works1/2
  Setpoint/1 -> Hand_Mode2/1
  [Enable_Auto] -> Hand_Mode2/2
  Constant2/1 -> Hand_Mode2/3
  Process_Value/1 -> Get_Current_Offset1/1(In1), Hand_Mode3/1
  [Enable_Auto] -> Hand_Mode3/2
  Constant3/1 -> Hand_Mode3/3
  Hand_Mode3/1 -> Substract Current Offset so that the linearised model works1/1
  Constant5/1 -> Hand_Mode4/3
  [Enable_Auto] -> Hand_Mode4/2
  Get_Current_Offset1/1(Hold when disabled) -> Hand_Mode4/1
  Time_Constant_System/1 -> PT1_Tustin/3(Time_Constant_System)
  Constant1/1 -> PT1_Tustin/2(Gain_System)
  Sample_Time/1 -> PT1_Tustin/4(Sample_Time)
  I_Controller/1 -> Check if Controller Integrator is 0/2, Invert Integrator/2
  Constant/1 -> Check if Controller Integrator is 0/3
  Invert Integrator/1 -> Check if Controller Integrator is 0/1
  Constant6/1 -> Invert Integrator/1
  Unit Delay/1 -> Sum/2
  [Enable_Auto] -> Scope/3, "PID Controller P multiply 1 plus Ti "/4
  Divide/1 -> "PID Controller P multiply 1 plus Ti "/5

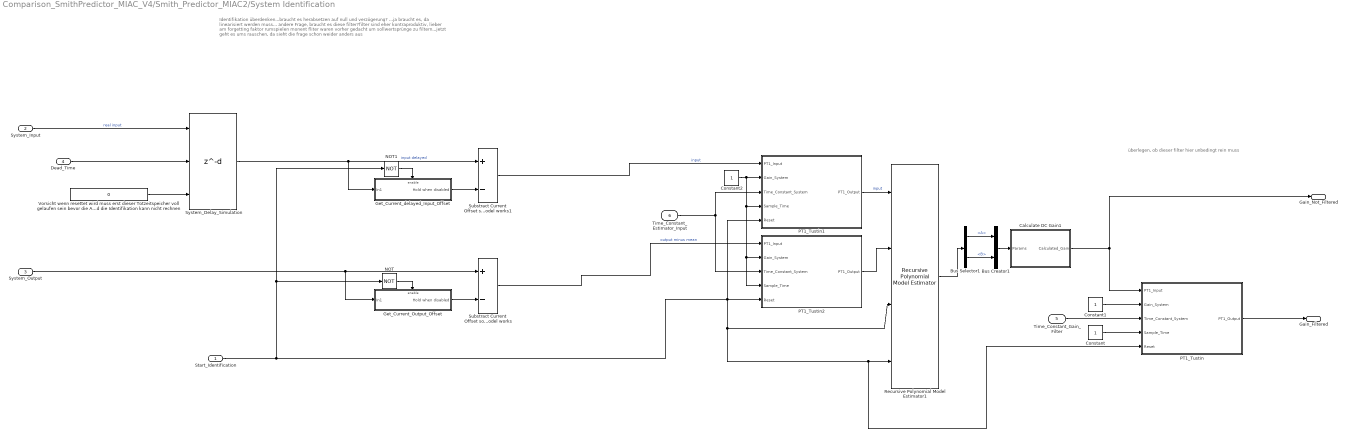
== system Comparison_SmithPredictor_MIAC_V4/Smith_Predictor_MIAC2/System Identification ==
  note: überlegen, ob dieser filter hier unbedingt rein muss
  note: Identifikation überdenken...braucht es herabsetzen auf null und verzögerung?
      | ...ja braucht es, da linearisiert werden muss...
      |
      | andere Frage, braucht es diese filter?filter sind eher kontraproduktiv, lieber am forgetting faktor rumspielen
      | monent fliter waren vorher gedacht um sollwertsprünge zu filtern...jetzt geht es ums rauschen, da sieht die frage schon weider anders aus
  Start_Identification : Inport  SampleTime=1
  System_Input : Inport  Port=2
  System_Output : Inport  Port=3  SampleTime=1
  Dead_Time : Inport  Port=4
  Time_Constant_Gain_Filter : Inport  Port=5
  Time_Constant_Estimator_Input : Inport  Port=6
  Bus Creator1 : BusCreator  Inputs=2
  Bus Selector1 : BusSelector  OutputSignals=A,B
  Calculate DC Gain1 : Subsystem  TreatAsAtomicUnit=on  SystemSampleTime=1
  Constant : Constant
  Constant1 : Constant
  Constant2 : Constant
  Get_Current_Output_Offset : Subsystem
  Get_Current_delayed_Input_Offset : Subsystem
  NOT : Logic  Operator=NOT  IconShape=distinctive  AllPortsSameDT=off  OutDataTypeStr=boolean
  NOT1 : Logic  Operator=NOT  IconShape=distinctive  AllPortsSameDT=off  OutDataTypeStr=boolean
  PT1_Tustin : Subsystem  TreatAsAtomicUnit=on  SystemSampleTime=1
  PT1_Tustin1 : Subsystem  TreatAsAtomicUnit=on  SystemSampleTime=1
  PT1_Tustin2 : Subsystem  TreatAsAtomicUnit=on  SystemSampleTime=1
  Recursive Polynomial Model Estimator1 : slident/Estimators/Recursive Polynomial Model Estimator  ModelStructure=ARX  InitialEstimateSource=None  A0=2  B0=1  C0=1  D0=1  F0=1  nk=1  P0=10  InitialInputs=0  InitialOutputs=0  History=Infinite  WindowLength=2000  EstimationMethod=Forgetting Factor  AdaptationParameter=1  HasTimeVaryingAdaptationParameter=off  NormalizationBias=eps  OutputError=off  OutputP=off  AddEnablePort=on  ExternalReset=Rising  InputProcessing=Sample-based  Ts=1
      settings: SourceProductName=System Identification Toolbox  SourceProductBaseCode=ID
  Substract Current Offset so that the linearised model works : Sum  Inputs=+-
  Substract Current Offset so that the linearised model works1 : Sum  Inputs=+-
  System_Delay_Simulation : Delay  DelayLengthSource=Input port  DelayLength=600  DelayLengthUpperLimit=800  ExternalReset=Rising  SampleTime=1
      settings: InputPortMap=u0,p1,r5
  Vorsicht wenn resettet wird muss erst dieser Totzeitspeicher voll gelaufen sein bevor die Adaption starten darf Sonst kommt heir immer 0 raus und die Identifikation kann nicht rechnen : Constant  Value=0
  Gain_Filtered : Outport
  Gain_Not_Filtered : Outport  Port=2
  wires:
  Recursive Polynomial Model Estimator1/1 -> Bus Selector1/1
  Substract Current Offset so that the linearised model works1/1 -> PT1_Tustin1/1(PT1_Input)  "input"
  Bus Creator1/1 -> Calculate DC Gain1/1(Params)
  Bus Selector1/1 -> Bus Creator1/1  "<A>"
  Bus Selector1/2 -> Bus Creator1/2  "<B>"
  Substract Current Offset so that the linearised model works/1 -> PT1_Tustin2/1(PT1_Input)  "output minus mean"
  NOT/1 -> Get_Current_Output_Offset/Enable
  Get_Current_Output_Offset/1(Hold when disabled) -> Substract Current Offset so that the linearised model works/2
  System_Output/1 -> Get_Current_Output_Offset/1(In1), Substract Current Offset so that the linearised model works/1
  Get_Current_delayed_Input_Offset/1(Hold when disabled) -> Substract Current Offset so that the linearised model works1/2
  NOT1/1 -> Get_Current_delayed_Input_Offset/Enable
  PT1_Tustin/1(PT1_Output) -> Gain_Filtered/1
  System_Input/1 -> System_Delay_Simulation/1  "real input"
  Vorsicht wenn resettet wird muss erst dieser Totzeitspeicher voll gelaufen sein bevor die Adaption starten darf Sonst kommt heir immer 0 raus und die Identifikation kann nicht rechnen/1 -> System_Delay_Simulation/3
  Dead_Time/1 -> System_Delay_Simulation/2
  System_Delay_Simulation/1 -> Substract Current Offset so that the linearised model works1/1, Get_Current_delayed_Input_Offset/1(In1)  "input delayed"
  Calculate DC Gain1/1(Calculated_Gain) -> PT1_Tustin/1(PT1_Input), Gain_Not_Filtered/1
  Start_Identification/1 -> NOT/1, NOT1/1, PT1_Tustin2/5(Reset), Recursive Polynomial Model Estimator1/3, PT1_Tustin/5(Reset), Recursive Polynomial Model Estimator1/4, PT1_Tustin1/5(Reset)
  Constant/1 -> PT1_Tustin/4(Sample_Time)
  Constant1/1 -> PT1_Tustin/2(Gain_System)
  Time_Constant_Gain_Filter/1 -> PT1_Tustin/3(Time_Constant_System)
  PT1_Tustin1/1(PT1_Output) -> Recursive Polynomial Model Estimator1/1  "input"
  PT1_Tustin2/1(PT1_Output) -> Recursive Polynomial Model Estimator1/2
  Constant2/1 -> PT1_Tustin1/2(Gain_System), PT1_Tustin2/2(Gain_System), PT1_Tustin2/4(Sample_Time), PT1_Tustin1/4(Sample_Time)
  Time_Constant_Estimator_Input/1 -> PT1_Tustin2/3(Time_Constant_System), PT1_Tustin1/3(Time_Constant_System)

== system Comparison_SmithPredictor_MIAC_V4/SmP_MIAC/Adaptive SmithPredictor1/Get_Current_Offset ==
  In1 : Inport
  Enable : EnablePort
  Hold when disabled : Outport
  wires:
  In1/1 -> Hold when disabled/1

== system Comparison_SmithPredictor_MIAC_V4/SmP_MIAC/Adaptive SmithPredictor1/Get_Current_Offset1 ==
  In1 : Inport
  Enable : EnablePort
  Hold when disabled : Outport
  wires:
  In1/1 -> Hold when disabled/1

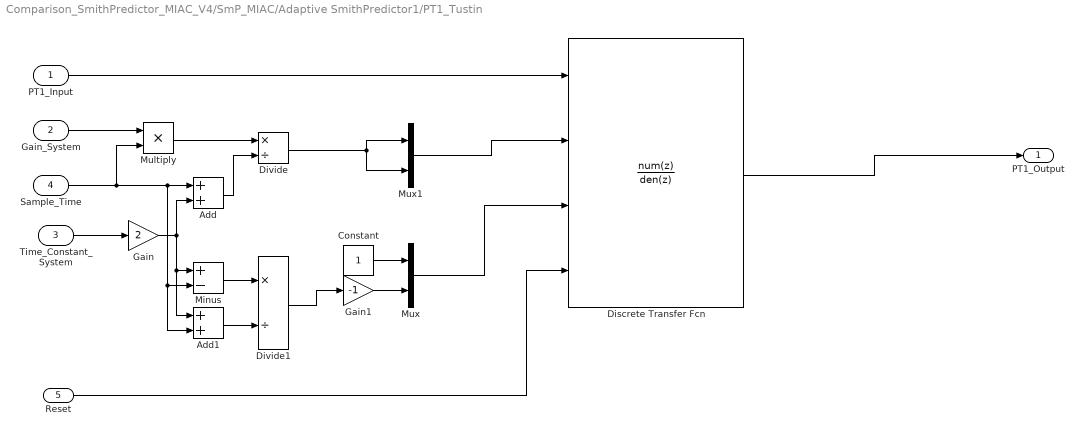
== system Comparison_SmithPredictor_MIAC_V4/SmP_MIAC/Adaptive SmithPredictor1/PT1_Tustin ==
  PT1_Input : Inport
  Gain_System : Inport  Port=2
  Time_Constant_System : Inport  Port=3
  Sample_Time : Inport  Port=4
  Reset : Inport  Port=5
  Add : Sum
  Add1 : Sum
  Constant : Constant
  Discrete Transfer Fcn : DiscreteTransferFcn  NumeratorSource=Input port  DenominatorSource=Input port  ExternalReset=Rising  SampleTime=1  a0EqualsOne=on
      settings: InputPortMap=u0,p1,p3,r7
  Divide : Product  Inputs=*/
  Divide1 : Product  Inputs=*/
  Gain : Gain  Gain=2
  Gain1 : Gain  Gain=-1
  Minus : Sum  Inputs=+-
  Multiply : Product
  Mux : Mux  Inputs=2
  Mux1 : Mux  Inputs=2
  PT1_Output : Outport
  wires:
  PT1_Input/1 -> Discrete Transfer Fcn/1
  Mux/1 -> Discrete Transfer Fcn/3
  Sample_Time/1 -> Add1/2, Minus/2, Add/1, Multiply/2
  Mux1/1 -> Discrete Transfer Fcn/2
  Time_Constant_System/1 -> Gain/1
  Discrete Transfer Fcn/1 -> PT1_Output/1
  Gain_System/1 -> Multiply/1
  Multiply/1 -> Divide/1
  Gain/1 -> Add1/1, Minus/1, Add/2
  Add/1 -> Divide/2
  Divide/1 -> Mux1/2, Mux1/1
  Constant/1 -> Mux/1
  Minus/1 -> Divide1/1
  Add1/1 -> Divide1/2
  Divide1/1 -> Gain1/1
  Gain1/1 -> Mux/2
  Reset/1 -> Discrete Transfer Fcn/4

== system Comparison_SmithPredictor_MIAC_V4/SmP_MIAC/System Identification/Calculate DC Gain1 ==
  Params : Inport
  A(z) Sum of Elements : Sum  Inputs=+
  B(z) Sum of Elements : Sum  Inputs=+
  Bus Selector : BusSelector  OutputSignals=B,A
  Divide : Product  Inputs=*/
  Gain_Saturation : Saturate  UpperLimit=1.5  LowerLimit=0.01
  Calculated_Gain : Outport
  wires:
  Params/1 -> Bus Selector/1
  Bus Selector/1 -> B(z) Sum of Elements/1  "<B>"
  Bus Selector/2 -> A(z) Sum of Elements/1  "<A>"
  B(z) Sum of Elements/1 -> Divide/1
  Divide/1 -> Gain_Saturation/1  "DCGain"
  A(z) Sum of Elements/1 -> Divide/2
  Gain_Saturation/1 -> Calculated_Gain/1

== system Comparison_SmithPredictor_MIAC_V4/SmP_MIAC/System Identification/Get_Current_Output_Offset ==
  In1 : Inport
  Enable : EnablePort
  Hold when disabled : Outport
  wires:
  In1/1 -> Hold when disabled/1

== system Comparison_SmithPredictor_MIAC_V4/SmP_MIAC/System Identification/Get_Current_delayed_Input_Offset ==
  In1 : Inport
  Enable : EnablePort
  Hold when disabled : Outport
  wires:
  In1/1 -> Hold when disabled/1

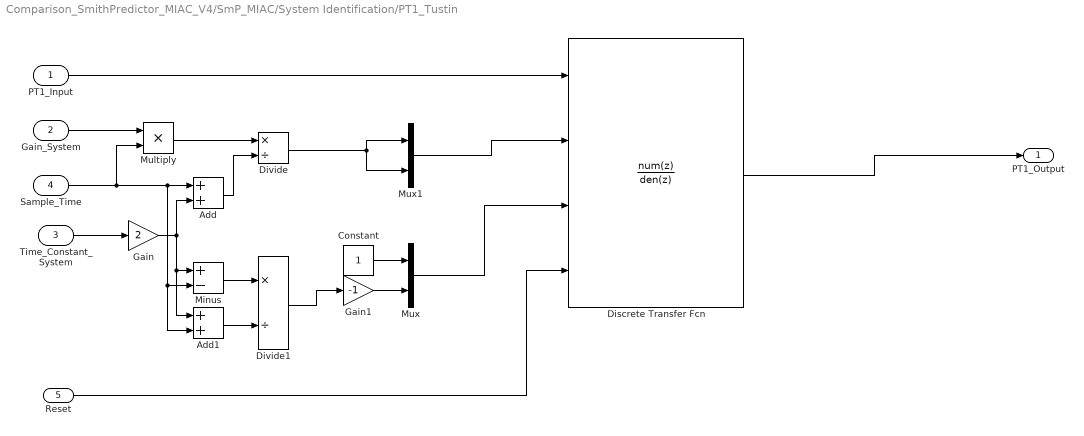
== system Comparison_SmithPredictor_MIAC_V4/SmP_MIAC/System Identification/PT1_Tustin ==
  PT1_Input : Inport
  Gain_System : Inport  Port=2
  Time_Constant_System : Inport  Port=3
  Sample_Time : Inport  Port=4
  Reset : Inport  Port=5
  Add : Sum
  Add1 : Sum
  Constant : Constant
  Discrete Transfer Fcn : DiscreteTransferFcn  NumeratorSource=Input port  DenominatorSource=Input port  ExternalReset=Rising  SampleTime=1  a0EqualsOne=on
      settings: InputPortMap=u0,p1,p3,r7
  Divide : Product  Inputs=*/
  Divide1 : Product  Inputs=*/
  Gain : Gain  Gain=2
  Gain1 : Gain  Gain=-1
  Minus : Sum  Inputs=+-
  Multiply : Product
  Mux : Mux  Inputs=2
  Mux1 : Mux  Inputs=2
  PT1_Output : Outport
  wires:
  PT1_Input/1 -> Discrete Transfer Fcn/1
  Mux/1 -> Discrete Transfer Fcn/3
  Sample_Time/1 -> Add1/2, Minus/2, Add/1, Multiply/2
  Mux1/1 -> Discrete Transfer Fcn/2
  Time_Constant_System/1 -> Gain/1
  Discrete Transfer Fcn/1 -> PT1_Output/1
  Gain_System/1 -> Multiply/1
  Multiply/1 -> Divide/1
  Gain/1 -> Add1/1, Minus/1, Add/2
  Add/1 -> Divide/2
  Divide/1 -> Mux1/2, Mux1/1
  Constant/1 -> Mux/1
  Minus/1 -> Divide1/1
  Add1/1 -> Divide1/2
  Divide1/1 -> Gain1/1
  Gain1/1 -> Mux/2
  Reset/1 -> Discrete Transfer Fcn/4

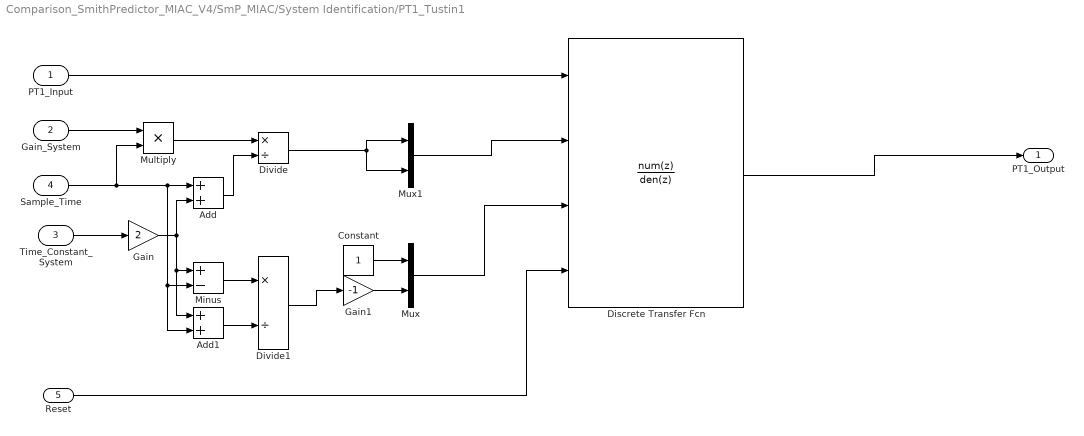
== system Comparison_SmithPredictor_MIAC_V4/SmP_MIAC/System Identification/PT1_Tustin1 ==
  PT1_Input : Inport
  Gain_System : Inport  Port=2
  Time_Constant_System : Inport  Port=3
  Sample_Time : Inport  Port=4
  Reset : Inport  Port=5
  Add : Sum
  Add1 : Sum
  Constant : Constant
  Discrete Transfer Fcn : DiscreteTransferFcn  NumeratorSource=Input port  DenominatorSource=Input port  ExternalReset=Rising  SampleTime=1  a0EqualsOne=on
      settings: InputPortMap=u0,p1,p3,r7
  Divide : Product  Inputs=*/
  Divide1 : Product  Inputs=*/
  Gain : Gain  Gain=2
  Gain1 : Gain  Gain=-1
  Minus : Sum  Inputs=+-
  Multiply : Product
  Mux : Mux  Inputs=2
  Mux1 : Mux  Inputs=2
  PT1_Output : Outport
  wires:
  PT1_Input/1 -> Discrete Transfer Fcn/1
  Mux/1 -> Discrete Transfer Fcn/3
  Sample_Time/1 -> Add1/2, Minus/2, Add/1, Multiply/2
  Mux1/1 -> Discrete Transfer Fcn/2
  Time_Constant_System/1 -> Gain/1
  Discrete Transfer Fcn/1 -> PT1_Output/1
  Gain_System/1 -> Multiply/1
  Multiply/1 -> Divide/1
  Gain/1 -> Add1/1, Minus/1, Add/2
  Add/1 -> Divide/2
  Divide/1 -> Mux1/2, Mux1/1
  Constant/1 -> Mux/1
  Minus/1 -> Divide1/1
  Add1/1 -> Divide1/2
  Divide1/1 -> Gain1/1
  Gain1/1 -> Mux/2
  Reset/1 -> Discrete Transfer Fcn/4

== system Comparison_SmithPredictor_MIAC_V4/SmP_MIAC/System Identification/PT1_Tustin2 ==
  PT1_Input : Inport
  Gain_System : Inport  Port=2
  Time_Constant_System : Inport  Port=3
  Sample_Time : Inport  Port=4
  Reset : Inport  Port=5
  Add : Sum
  Add1 : Sum
  Constant : Constant
  Discrete Transfer Fcn : DiscreteTransferFcn  NumeratorSource=Input port  DenominatorSource=Input port  ExternalReset=Rising  SampleTime=1  a0EqualsOne=on
      settings: InputPortMap=u0,p1,p3,r7
  Divide : Product  Inputs=*/
  Divide1 : Product  Inputs=*/
  Gain : Gain  Gain=2
  Gain1 : Gain  Gain=-1
  Minus : Sum  Inputs=+-
  Multiply : Product
  Mux : Mux  Inputs=2
  Mux1 : Mux  Inputs=2
  PT1_Output : Outport
  wires:
  PT1_Input/1 -> Discrete Transfer Fcn/1
  Mux/1 -> Discrete Transfer Fcn/3
  Sample_Time/1 -> Add1/2, Minus/2, Add/1, Multiply/2
  Mux1/1 -> Discrete Transfer Fcn/2
  Time_Constant_System/1 -> Gain/1
  Discrete Transfer Fcn/1 -> PT1_Output/1
  Gain_System/1 -> Multiply/1
  Multiply/1 -> Divide/1
  Gain/1 -> Add1/1, Minus/1, Add/2
  Add/1 -> Divide/2
  Divide/1 -> Mux1/2, Mux1/1
  Constant/1 -> Mux/1
  Minus/1 -> Divide1/1
  Add1/1 -> Divide1/2
  Divide1/1 -> Gain1/1
  Gain1/1 -> Mux/2
  Reset/1 -> Discrete Transfer Fcn/4

== system Comparison_SmithPredictor_MIAC_V4/Smith_Predictor_MIAC2/Adaptive SmithPredictor1/Get_Current_Offset ==
  In1 : Inport
  Enable : EnablePort
  Hold when disabled : Outport
  wires:
  In1/1 -> Hold when disabled/1

== system Comparison_SmithPredictor_MIAC_V4/Smith_Predictor_MIAC2/Adaptive SmithPredictor1/Get_Current_Offset1 ==
  In1 : Inport
  Enable : EnablePort
  Hold when disabled : Outport
  wires:
  In1/1 -> Hold when disabled/1

== system Comparison_SmithPredictor_MIAC_V4/Smith_Predictor_MIAC2/Adaptive SmithPredictor1/PT1_Tustin ==
  PT1_Input : Inport
  Gain_System : Inport  Port=2
  Time_Constant_System : Inport  Port=3
  Sample_Time : Inport  Port=4
  Reset : Inport  Port=5
  Add : Sum
  Add1 : Sum
  Constant : Constant
  Discrete Transfer Fcn : DiscreteTransferFcn  NumeratorSource=Input port  DenominatorSource=Input port  ExternalReset=Rising  SampleTime=1  a0EqualsOne=on
      settings: InputPortMap=u0,p1,p3,r7
  Divide : Product  Inputs=*/
  Divide1 : Product  Inputs=*/
  Gain : Gain  Gain=2
  Gain1 : Gain  Gain=-1
  Minus : Sum  Inputs=+-
  Multiply : Product
  Mux : Mux  Inputs=2
  Mux1 : Mux  Inputs=2
  PT1_Output : Outport
  wires:
  PT1_Input/1 -> Discrete Transfer Fcn/1
  Mux/1 -> Discrete Transfer Fcn/3
  Sample_Time/1 -> Add1/2, Minus/2, Add/1, Multiply/2
  Mux1/1 -> Discrete Transfer Fcn/2
  Time_Constant_System/1 -> Gain/1
  Discrete Transfer Fcn/1 -> PT1_Output/1
  Gain_System/1 -> Multiply/1
  Multiply/1 -> Divide/1
  Gain/1 -> Add1/1, Minus/1, Add/2
  Add/1 -> Divide/2
  Divide/1 -> Mux1/2, Mux1/1
  Constant/1 -> Mux/1
  Minus/1 -> Divide1/1
  Add1/1 -> Divide1/2
  Divide1/1 -> Gain1/1
  Gain1/1 -> Mux/2
  Reset/1 -> Discrete Transfer Fcn/4

== system Comparison_SmithPredictor_MIAC_V4/Smith_Predictor_MIAC2/System Identification/Calculate DC Gain1 ==
  Params : Inport
  A(z) Sum of Elements : Sum  Inputs=+
  B(z) Sum of Elements : Sum  Inputs=+
  Bus Selector : BusSelector  OutputSignals=B,A
  Divide : Product  Inputs=*/
  Gain_Saturation : Saturate  UpperLimit=1.5  LowerLimit=0.01
  Calculated_Gain : Outport
  wires:
  Params/1 -> Bus Selector/1
  Bus Selector/1 -> B(z) Sum of Elements/1  "<B>"
  Bus Selector/2 -> A(z) Sum of Elements/1  "<A>"
  B(z) Sum of Elements/1 -> Divide/1
  Divide/1 -> Gain_Saturation/1  "DCGain"
  A(z) Sum of Elements/1 -> Divide/2
  Gain_Saturation/1 -> Calculated_Gain/1

== system Comparison_SmithPredictor_MIAC_V4/Smith_Predictor_MIAC2/System Identification/Get_Current_Output_Offset ==
  In1 : Inport
  Enable : EnablePort
  Hold when disabled : Outport
  wires:
  In1/1 -> Hold when disabled/1

== system Comparison_SmithPredictor_MIAC_V4/Smith_Predictor_MIAC2/System Identification/Get_Current_delayed_Input_Offset ==
  In1 : Inport
  Enable : EnablePort
  Hold when disabled : Outport
  wires:
  In1/1 -> Hold when disabled/1

== system Comparison_SmithPredictor_MIAC_V4/Smith_Predictor_MIAC2/System Identification/PT1_Tustin ==
  PT1_Input : Inport
  Gain_System : Inport  Port=2
  Time_Constant_System : Inport  Port=3
  Sample_Time : Inport  Port=4
  Reset : Inport  Port=5
  Add : Sum
  Add1 : Sum
  Constant : Constant
  Discrete Transfer Fcn : DiscreteTransferFcn  NumeratorSource=Input port  DenominatorSource=Input port  ExternalReset=Rising  SampleTime=1  a0EqualsOne=on
      settings: InputPortMap=u0,p1,p3,r7
  Divide : Product  Inputs=*/
  Divide1 : Product  Inputs=*/
  Gain : Gain  Gain=2
  Gain1 : Gain  Gain=-1
  Minus : Sum  Inputs=+-
  Multiply : Product
  Mux : Mux  Inputs=2
  Mux1 : Mux  Inputs=2
  PT1_Output : Outport
  wires:
  PT1_Input/1 -> Discrete Transfer Fcn/1
  Mux/1 -> Discrete Transfer Fcn/3
  Sample_Time/1 -> Add1/2, Minus/2, Add/1, Multiply/2
  Mux1/1 -> Discrete Transfer Fcn/2
  Time_Constant_System/1 -> Gain/1
  Discrete Transfer Fcn/1 -> PT1_Output/1
  Gain_System/1 -> Multiply/1
  Multiply/1 -> Divide/1
  Gain/1 -> Add1/1, Minus/1, Add/2
  Add/1 -> Divide/2
  Divide/1 -> Mux1/2, Mux1/1
  Constant/1 -> Mux/1
  Minus/1 -> Divide1/1
  Add1/1 -> Divide1/2
  Divide1/1 -> Gain1/1
  Gain1/1 -> Mux/2
  Reset/1 -> Discrete Transfer Fcn/4

== system Comparison_SmithPredictor_MIAC_V4/Smith_Predictor_MIAC2/System Identification/PT1_Tustin1 ==
  PT1_Input : Inport
  Gain_System : Inport  Port=2
  Time_Constant_System : Inport  Port=3
  Sample_Time : Inport  Port=4
  Reset : Inport  Port=5
  Add : Sum
  Add1 : Sum
  Constant : Constant
  Discrete Transfer Fcn : DiscreteTransferFcn  NumeratorSource=Input port  DenominatorSource=Input port  ExternalReset=Rising  SampleTime=1  a0EqualsOne=on
      settings: InputPortMap=u0,p1,p3,r7
  Divide : Product  Inputs=*/
  Divide1 : Product  Inputs=*/
  Gain : Gain  Gain=2
  Gain1 : Gain  Gain=-1
  Minus : Sum  Inputs=+-
  Multiply : Product
  Mux : Mux  Inputs=2
  Mux1 : Mux  Inputs=2
  PT1_Output : Outport
  wires:
  PT1_Input/1 -> Discrete Transfer Fcn/1
  Mux/1 -> Discrete Transfer Fcn/3
  Sample_Time/1 -> Add1/2, Minus/2, Add/1, Multiply/2
  Mux1/1 -> Discrete Transfer Fcn/2
  Time_Constant_System/1 -> Gain/1
  Discrete Transfer Fcn/1 -> PT1_Output/1
  Gain_System/1 -> Multiply/1
  Multiply/1 -> Divide/1
  Gain/1 -> Add1/1, Minus/1, Add/2
  Add/1 -> Divide/2
  Divide/1 -> Mux1/2, Mux1/1
  Constant/1 -> Mux/1
  Minus/1 -> Divide1/1
  Add1/1 -> Divide1/2
  Divide1/1 -> Gain1/1
  Gain1/1 -> Mux/2
  Reset/1 -> Discrete Transfer Fcn/4

== system Comparison_SmithPredictor_MIAC_V4/Smith_Predictor_MIAC2/System Identification/PT1_Tustin2 ==
  PT1_Input : Inport
  Gain_System : Inport  Port=2
  Time_Constant_System : Inport  Port=3
  Sample_Time : Inport  Port=4
  Reset : Inport  Port=5
  Add : Sum
  Add1 : Sum
  Constant : Constant
  Discrete Transfer Fcn : DiscreteTransferFcn  NumeratorSource=Input port  DenominatorSource=Input port  ExternalReset=Rising  SampleTime=1  a0EqualsOne=on
      settings: InputPortMap=u0,p1,p3,r7
  Divide : Product  Inputs=*/
  Divide1 : Product  Inputs=*/
  Gain : Gain  Gain=2
  Gain1 : Gain  Gain=-1
  Minus : Sum  Inputs=+-
  Multiply : Product
  Mux : Mux  Inputs=2
  Mux1 : Mux  Inputs=2
  PT1_Output : Outport
  wires:
  PT1_Input/1 -> Discrete Transfer Fcn/1
  Mux/1 -> Discrete Transfer Fcn/3
  Sample_Time/1 -> Add1/2, Minus/2, Add/1, Multiply/2
  Mux1/1 -> Discrete Transfer Fcn/2
  Time_Constant_System/1 -> Gain/1
  Discrete Transfer Fcn/1 -> PT1_Output/1
  Gain_System/1 -> Multiply/1
  Multiply/1 -> Divide/1
  Gain/1 -> Add1/1, Minus/1, Add/2
  Add/1 -> Divide/2
  Divide/1 -> Mux1/2, Mux1/1
  Constant/1 -> Mux/1
  Minus/1 -> Divide1/1
  Add1/1 -> Divide1/2
  Divide1/1 -> Gain1/1
  Gain1/1 -> Mux/2
  Reset/1 -> Discrete Transfer Fcn/4
